simulink model "sample_trajectory"  (R2014a)
settings: Solver=ode3  StartTime=0.0  StopTime=2*apex_time  FixedStep=0.001  MaxStep=1e-2  RelTol=1e-3  AbsTol=1e-4
undefined symbols (not defined in the file or in its folder): alpha_apex, apex_time, d_y_com, l0_virtual, max_leg_length, min_leg_length
libraries: simulink x10
settings Model: Creator=wmartin  LastModifiedBy=wmartin

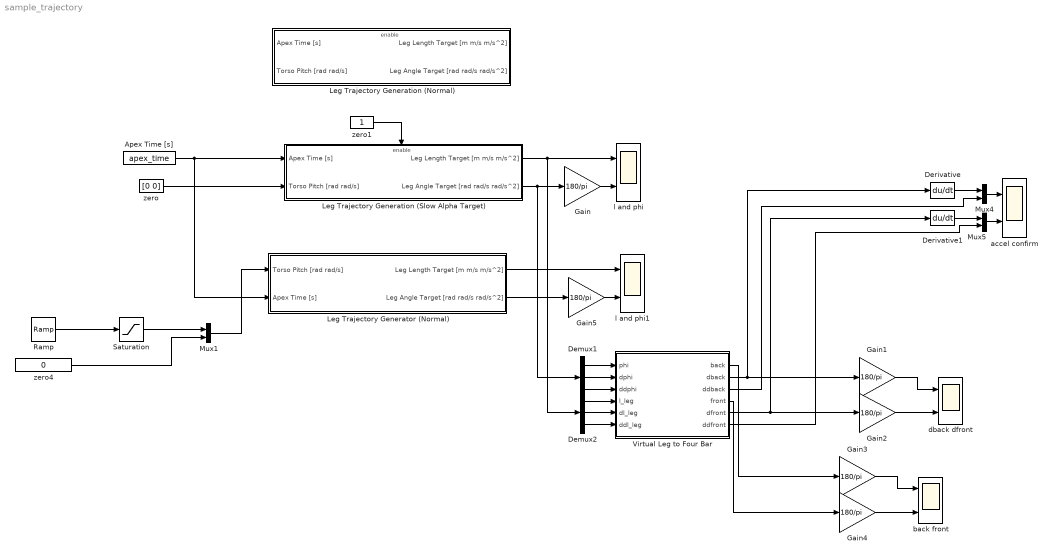
== system sample_trajectory ==
  Apex Time [s] : Constant  Value=apex_time
  Demux1 : Demux  Outputs=3
  Demux2 : Demux  Outputs=3
  Derivative : Derivative
  Derivative1 : Derivative
  Gain{,1..5} (6 alike) : Gain  Gain=180/pi
  Leg Trajectory Generation (Normal) : Subsystem
  Leg Trajectory Generation (Slow Alpha Target) : Subsystem
  Leg Trajectory Generator (Normal) : Subsystem
  Mux1 : Mux  Inputs=2
  Mux4 : Mux  Inputs=2
  Mux5 : Mux  Inputs=2
  Ramp : simulink/Sources/Ramp  slope=-20*pi/180 / apex_time  start=0  X0=0
  Saturation : Saturate  UpperLimit=20*pi/180  LowerLimit=-20*pi/180
  Virtual Leg to Four Bar : MATLAB Function  TreatAsAtomicUnit=on
  accel confirm : Scope  NumInputPorts=2
      settings: YMin=-5~-5  YMax=5~5  SaveName=ScopeData3
  back front : Scope  NumInputPorts=2
      settings: YMin=-5~-5  YMax=5~5  SaveName=ScopeData4
  dback dfront : Scope  NumInputPorts=2
      settings: YMin=-5~-5  YMax=5~5
  l and phi : Scope  NumInputPorts=2
      settings: YMin=-5~-5  YMax=5~5  SaveName=ScopeData2
  l and phi1 : Scope  NumInputPorts=2
      settings: YMin=-35~-3500  YMax=40~4000  SaveName=ScopeData5
  zero : Constant  Value=[0 0]
  zero1 : Constant
  zero4 : Constant  Value=0
  wires:
  Gain/1 -> l and phi/2
  Leg Trajectory Generation (Slow Alpha Target)/2(Leg Angle Target [rad rad/s rad/s^2]) -> Demux1/1, Gain/1
  Apex Time [s]/1 -> Leg Trajectory Generator (Normal)/2(Apex Time [s]), Leg Trajectory Generation (Slow Alpha Target)/1(Apex Time [s])
  Leg Trajectory Generation (Slow Alpha Target)/1(Leg Length Target [m m/s m/s^2]) -> Demux2/1, l and phi/1
  Demux1/1 -> Virtual Leg to Four Bar/1(phi)
  Demux1/2 -> Virtual Leg to Four Bar/2(dphi)
  Demux2/1 -> Virtual Leg to Four Bar/4(l_leg)
  Demux2/2 -> Virtual Leg to Four Bar/5(dl_leg)
  Gain1/1 -> dback dfront/1
  Gain2/1 -> dback dfront/2
  Virtual Leg to Four Bar/3(ddback) -> Mux4/2
  Virtual Leg to Four Bar/5(dfront) -> Derivative1/1, Gain2/1
  Virtual Leg to Four Bar/6(ddfront) -> Mux5/2
  Virtual Leg to Four Bar/2(dback) -> Derivative/1, Gain1/1
  Derivative/1 -> Mux4/1
  Mux4/1 -> accel confirm/1
  Derivative1/1 -> Mux5/1
  Mux5/1 -> accel confirm/2
  Demux1/3 -> Virtual Leg to Four Bar/3(ddphi)
  Demux2/3 -> Virtual Leg to Four Bar/6(ddl_leg)
  Gain3/1 -> back front/1
  Gain4/1 -> back front/2
  Virtual Leg to Four Bar/1(back) -> Gain3/1
  Virtual Leg to Four Bar/4(front) -> Gain4/1
  zero1/1 -> Leg Trajectory Generation (Slow Alpha Target)/Enable
  Gain5/1 -> l and phi1/2
  Leg Trajectory Generator (Normal)/1(Leg Length Target [m m/s m/s^2]) -> l and phi1/1
  Leg Trajectory Generator (Normal)/2(Leg Angle Target [rad rad/s rad/s^2]) -> Gain5/1
  zero/1 -> Leg Trajectory Generation (Slow Alpha Target)/2(Torso Pitch [rad rad/s])
  zero4/1 -> Mux1/2
  Mux1/1 -> Leg Trajectory Generator (Normal)/1(Torso Pitch [rad rad/s])
  Ramp/1 -> Saturation/1
  Saturation/1 -> Mux1/1

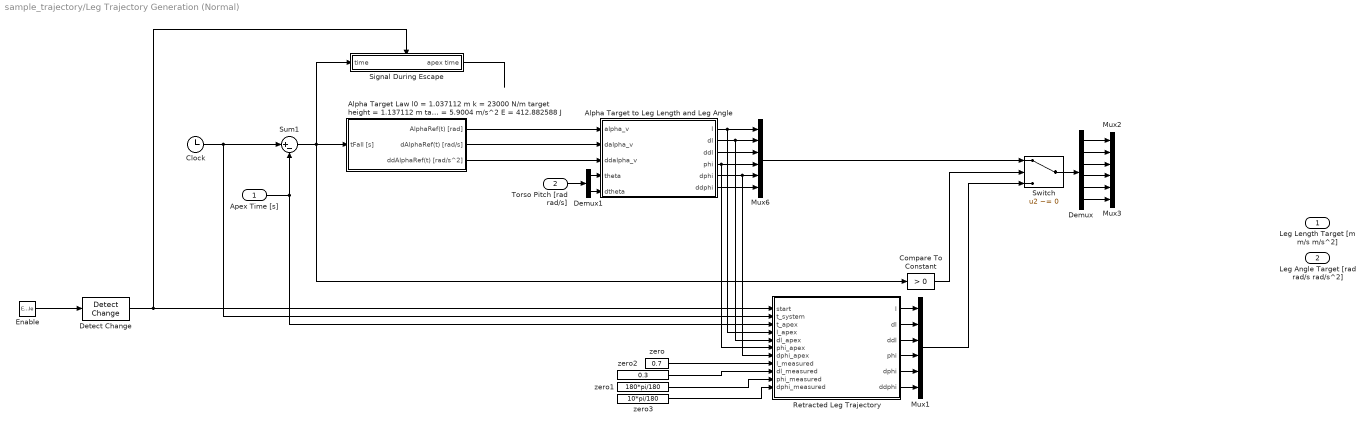
== system sample_trajectory/Leg Trajectory Generation (Normal) ==
  Apex Time [s] : Inport
  Torso Pitch [rad rad/s] : Inport  Port=2
  Enable : EnablePort  StatesWhenEnabling=reset  ShowOutputPort=on  ZeroCross=off
      settings: AttributesFormatString=When enabled: %<StatesWhenEnabling>
  Alpha Target Law l0 = 1.037112 m k = 23000 N/m target height = 1.137112 m target speed = 0.5 m/s m = 60.4120 kg g = 5.9004 m/s^2 E = 412.882588 J : Subsystem
  Alpha Target to Leg Length and Leg Angle : MATLAB Function  TreatAsAtomicUnit=on
  Clock : Clock
  Compare To Constant : simulink/Logic and Bit Operations/Compare To Constant  relop=>  const=0  OutDataTypeStr=boolean  ZeroCross=off
  Demux : Demux  Outputs=6
  Demux1 : Demux  Outputs=2
  Detect Change : simulink/Logic and Bit Operations/Detect Change  vinit=0  InputProcessing=Inherited  OutDataTypeStr=boolean
  Mux1 : Mux  Inputs=6
  Mux2 : Mux  Inputs=3
  Mux3 : Mux  Inputs=3
  Mux6 : Mux  Inputs=6
  Retracted Leg Trajectory : MATLAB Function  TreatAsAtomicUnit=on
  Signal During Escape : Subsystem
  Sum1 : Sum  Inputs=|+-
  Switch : Switch  Criteria=u2 ~= 0
  zero : Constant  Value=0.7
  zero1 : Constant  Value=180*pi/180
  zero2 : Constant  Value=0.3
  zero3 : Constant  Value=10*pi/180
  Leg Length Target [m m/s m/s^2] : Outport
  Leg Angle Target [rad rad/s rad/s^2] : Outport  Port=2
  wires:
  Signal During Escape/1(apex time) -> ?
  Clock/1 -> Sum1/1, Retracted Leg Trajectory/2(t_system)
  zero3/1 -> Retracted Leg Trajectory/11(dphi_measured)
  zero1/1 -> Retracted Leg Trajectory/10(phi_measured)
  zero2/1 -> Retracted Leg Trajectory/9(dl_measured)
  zero/1 -> Retracted Leg Trajectory/8(l_measured)
  Torso Pitch [rad rad/s]/1 -> Demux1/1
  Mux1/1 -> Switch/3
  Compare To Constant/1 -> Switch/2
  Apex Time [s]/1 -> Sum1/2, Retracted Leg Trajectory/3(t_apex)
  Alpha Target Law l0 = 1.037112 m k = 23000 N/m target height = 1.137112 m target speed = 0.5 m/s m = 60.4120 kg g = 5.9004 m/s^2 E = 412.882588 J/1(AlphaRef(t) [rad]) -> Alpha Target to Leg Length and Leg Angle/1(alpha_v)
  Sum1/1 -> Compare To Constant/1, Alpha Target Law l0 = 1.037112 m k = 23000 N/m target height = 1.137112 m target speed = 0.5 m/s m = 60.4120 kg g = 5.9004 m/s^2 E = 412.882588 J/1(tFall [s]), Signal During Escape/1(time)
  Retracted Leg Trajectory/1(l) -> Mux1/1
  Retracted Leg Trajectory/4(phi) -> Mux1/4
  Retracted Leg Trajectory/2(dl) -> Mux1/2
  Retracted Leg Trajectory/5(dphi) -> Mux1/5
  Enable/1 -> Detect Change/1
  Detect Change/1 -> Retracted Leg Trajectory/1(start), Signal During Escape/Enable
  Alpha Target to Leg Length and Leg Angle/4(phi) -> Mux6/4, Retracted Leg Trajectory/6(phi_apex)
  Alpha Target to Leg Length and Leg Angle/3(ddl) -> Mux6/3
  Alpha Target to Leg Length and Leg Angle/5(dphi) -> Mux6/5, Retracted Leg Trajectory/7(dphi_apex)
  Alpha Target to Leg Length and Leg Angle/6(ddphi) -> Mux6/6
  Alpha Target to Leg Length and Leg Angle/2(dl) -> Mux6/2, Retracted Leg Trajectory/5(dl_apex)
  Alpha Target to Leg Length and Leg Angle/1(l) -> Mux6/1, Retracted Leg Trajectory/4(l_apex)
  Switch/1 -> Demux/1
  Demux/6 -> Mux3/3
  Demux/5 -> Mux3/2
  Demux/4 -> Mux3/1
  Demux/3 -> Mux2/3
  Demux/2 -> Mux2/2
  Demux/1 -> Mux2/1
  Demux1/1 -> Alpha Target to Leg Length and Leg Angle/4(theta)
  Demux1/2 -> Alpha Target to Leg Length and Leg Angle/5(dtheta)
  Mux6/1 -> Switch/1
  Alpha Target Law l0 = 1.037112 m k = 23000 N/m target height = 1.137112 m target speed = 0.5 m/s m = 60.4120 kg g = 5.9004 m/s^2 E = 412.882588 J/3(ddAlphaRef(t) [rad/s^2]) -> Alpha Target to Leg Length and Leg Angle/3(ddalpha_v)
  Alpha Target Law l0 = 1.037112 m k = 23000 N/m target height = 1.137112 m target speed = 0.5 m/s m = 60.4120 kg g = 5.9004 m/s^2 E = 412.882588 J/2(dAlphaRef(t) [rad/s]) -> Alpha Target to Leg Length and Leg Angle/2(dalpha_v)
  Retracted Leg Trajectory/3(ddl) -> Mux1/3
  Retracted Leg Trajectory/6(ddphi) -> Mux1/6

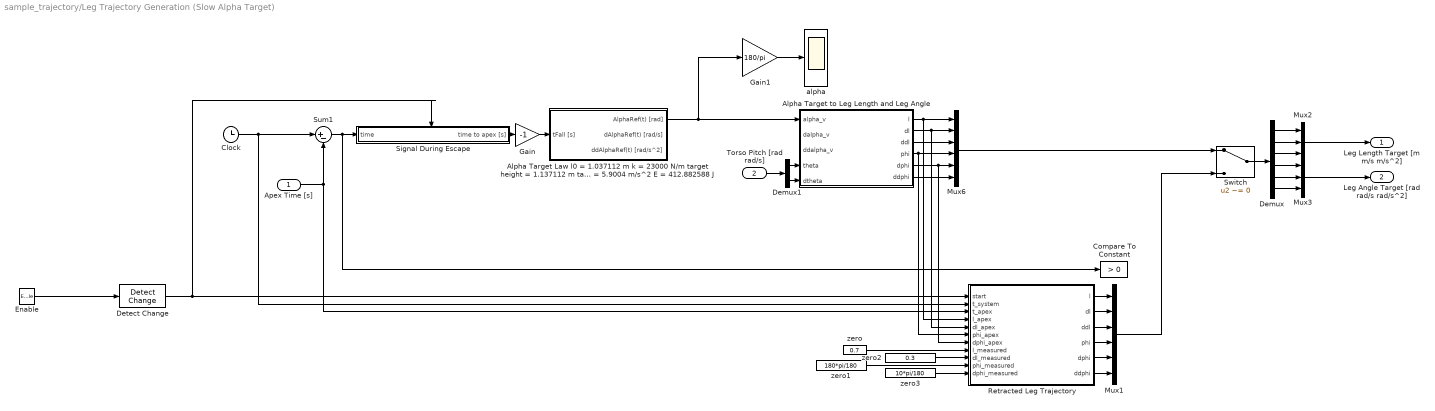
== system sample_trajectory/Leg Trajectory Generation (Slow Alpha Target) ==
  Apex Time [s] : Inport
  Torso Pitch [rad rad/s] : Inport  Port=2
  Enable : EnablePort  StatesWhenEnabling=reset  ShowOutputPort=on  ZeroCross=off
      settings: AttributesFormatString=When enabled: %<StatesWhenEnabling>
  Alpha Target Law l0 = 1.037112 m k = 23000 N/m target height = 1.137112 m target speed = 0.5 m/s m = 60.4120 kg g = 5.9004 m/s^2 E = 412.882588 J : Subsystem
  Alpha Target to Leg Length and Leg Angle : MATLAB Function  TreatAsAtomicUnit=on
  Clock : Clock
  Compare To Constant : simulink/Logic and Bit Operations/Compare To Constant  relop=>  const=0  OutDataTypeStr=boolean  ZeroCross=off
  Demux : Demux  Outputs=6
  Demux1 : Demux  Outputs=2
  Detect Change : simulink/Logic and Bit Operations/Detect Change  vinit=0  InputProcessing=Inherited  OutDataTypeStr=boolean
  Gain : Gain  Gain=-1
  Gain1 : Gain  Gain=180/pi
  Mux1 : Mux  Inputs=6
  Mux2 : Mux  Inputs=3
  Mux3 : Mux  Inputs=3
  Mux6 : Mux  Inputs=6
  Retracted Leg Trajectory : MATLAB Function  TreatAsAtomicUnit=on
  Signal During Escape : Subsystem
  Sum1 : Sum  Inputs=|+-
  Switch : Switch  Criteria=u2 ~= 0
  alpha : Scope
  zero : Constant  Value=0.7
  zero1 : Constant  Value=180*pi/180
  zero2 : Constant  Value=0.3
  zero3 : Constant  Value=10*pi/180
  Leg Length Target [m m/s m/s^2] : Outport
  Leg Angle Target [rad rad/s rad/s^2] : Outport  Port=2
  wires:
  Retracted Leg Trajectory/6(ddphi) -> Mux1/6
  Retracted Leg Trajectory/3(ddl) -> Mux1/3
  Mux6/1 -> Switch/1
  Demux1/2 -> Alpha Target to Leg Length and Leg Angle/5(dtheta)
  Demux1/1 -> Alpha Target to Leg Length and Leg Angle/4(theta)
  Demux/1 -> Mux2/1
  Demux/2 -> Mux2/2
  Demux/3 -> Mux2/3
  Demux/4 -> Mux3/1
  Demux/5 -> Mux3/2
  Demux/6 -> Mux3/3
  Switch/1 -> Demux/1
  Alpha Target to Leg Length and Leg Angle/1(l) -> Retracted Leg Trajectory/4(l_apex), Mux6/1
  Alpha Target to Leg Length and Leg Angle/2(dl) -> Retracted Leg Trajectory/5(dl_apex), Mux6/2
  Alpha Target to Leg Length and Leg Angle/6(ddphi) -> Mux6/6
  Alpha Target to Leg Length and Leg Angle/5(dphi) -> Retracted Leg Trajectory/7(dphi_apex), Mux6/5
  Alpha Target to Leg Length and Leg Angle/3(ddl) -> Mux6/3
  Alpha Target to Leg Length and Leg Angle/4(phi) -> Retracted Leg Trajectory/6(phi_apex), Mux6/4
  Detect Change/1 -> Retracted Leg Trajectory/1(start), Signal During Escape/Enable
  Apex Time [s]/1 -> Retracted Leg Trajectory/3(t_apex), Sum1/2
  Retracted Leg Trajectory/5(dphi) -> Mux1/5
  Retracted Leg Trajectory/2(dl) -> Mux1/2
  Retracted Leg Trajectory/4(phi) -> Mux1/4
  Retracted Leg Trajectory/1(l) -> Mux1/1
  Sum1/1 -> Signal During Escape/1(time), Compare To Constant/1
  Alpha Target Law l0 = 1.037112 m k = 23000 N/m target height = 1.137112 m target speed = 0.5 m/s m = 60.4120 kg g = 5.9004 m/s^2 E = 412.882588 J/1(AlphaRef(t) [rad]) -> Gain1/1, Alpha Target to Leg Length and Leg Angle/1(alpha_v)
  Mux1/1 -> Switch/3
  Torso Pitch [rad rad/s]/1 -> Demux1/1
  zero/1 -> Retracted Leg Trajectory/8(l_measured)
  zero2/1 -> Retracted Leg Trajectory/9(dl_measured)
  zero1/1 -> Retracted Leg Trajectory/10(phi_measured)
  zero3/1 -> Retracted Leg Trajectory/11(dphi_measured)
  Clock/1 -> Retracted Leg Trajectory/2(t_system), Sum1/1
  Signal During Escape/1(time to apex [s]) -> Gain/1
  Gain/1 -> Alpha Target Law l0 = 1.037112 m k = 23000 N/m target height = 1.137112 m target speed = 0.5 m/s m = 60.4120 kg g = 5.9004 m/s^2 E = 412.882588 J/1(tFall [s])
  Mux2/1 -> Leg Length Target [m m/s m/s^2]/1
  Mux3/1 -> Leg Angle Target [rad rad/s rad/s^2]/1
  Enable/1 -> Detect Change/1
  Gain1/1 -> alpha/1

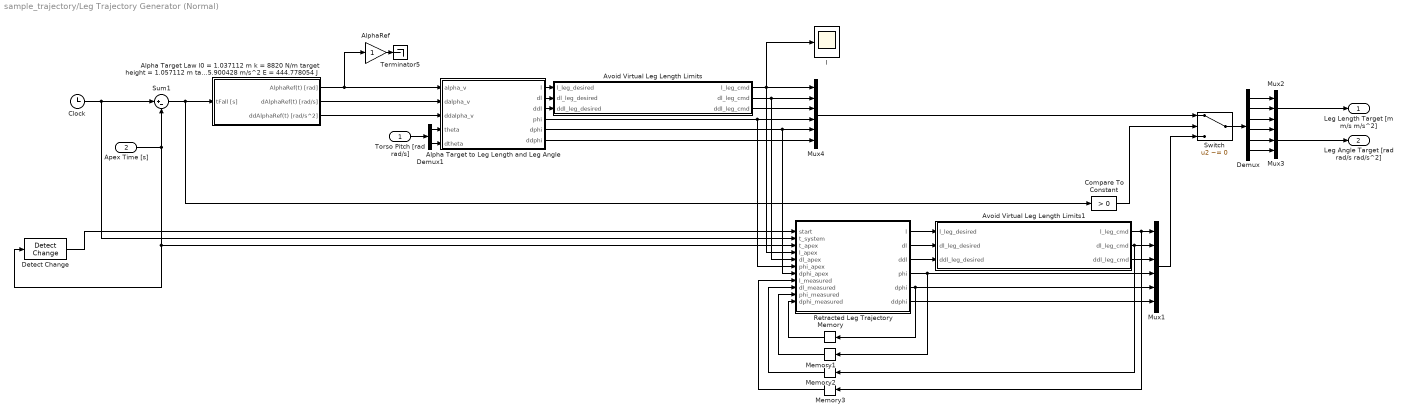
== system sample_trajectory/Leg Trajectory Generator (Normal) ==
  Torso Pitch [rad rad/s] : Inport
  Apex Time [s] : Inport  Port=2
  Alpha Target Law l0 = 1.037112 m k = 8820 N/m target height = 1.057112 m target speed = 1.0 m/s m = 60.4120 kg g = 5.900428 m/s^2 E = 444.778054 J : Subsystem
  Alpha Target to Leg Length and Leg Angle : MATLAB Function  TreatAsAtomicUnit=on
  AlphaRef : Gain
  Avoid Virtual Leg Length Limits : MATLAB Function  TreatAsAtomicUnit=on
  Avoid Virtual Leg Length Limits1 : MATLAB Function  TreatAsAtomicUnit=on
  Clock : Clock
  Compare To Constant : simulink/Logic and Bit Operations/Compare To Constant  relop=>  const=0  OutDataTypeStr=boolean  ZeroCross=off
  Demux : Demux  Outputs=6
  Demux1 : Demux  Outputs=2
  Detect Change : simulink/Logic and Bit Operations/Detect Change  vinit=0  InputProcessing=Inherited  OutDataTypeStr=boolean
  Memory : Memory  X0=-10*pi/180
  Memory1 : Memory  X0=159.2*pi/180
  Memory2 : Memory  X0=0.3
  Memory3 : Memory  X0=0.7738
  Mux1 : Mux  Inputs=6
  Mux2 : Mux  Inputs=3
  Mux3 : Mux  Inputs=3
  Mux4 : Mux  Inputs=6
  Retracted Leg Trajectory : MATLAB Function  TreatAsAtomicUnit=on
  Sum1 : Sum  Inputs=|+-
  Switch : Switch  Criteria=u2 ~= 0
  Terminator5 : Terminator
  l : Scope
      settings: SaveName=ScopeData6
  Leg Length Target [m m/s m/s^2] : Outport
  Leg Angle Target [rad rad/s rad/s^2] : Outport  Port=2
  wires:
  Torso Pitch [rad rad/s]/1 -> Demux1/1
  Mux1/1 -> Switch/3
  Compare To Constant/1 -> Switch/2
  Apex Time [s]/1 -> Detect Change/1, Retracted Leg Trajectory/3(t_apex), Sum1/2
  Clock/1 -> Retracted Leg Trajectory/2(t_system), Sum1/1
  Alpha Target Law l0 = 1.037112 m k = 8820 N/m target height = 1.057112 m target speed = 1.0 m/s m = 60.4120 kg g = 5.900428 m/s^2 E = 444.778054 J/1(AlphaRef(t) [rad]) -> AlphaRef/1, Alpha Target to Leg Length and Leg Angle/1(alpha_v)
  Sum1/1 -> Alpha Target Law l0 = 1.037112 m k = 8820 N/m target height = 1.057112 m target speed = 1.0 m/s m = 60.4120 kg g = 5.900428 m/s^2 E = 444.778054 J/1(tFall [s]), Compare To Constant/1
  AlphaRef/1 -> Terminator5/1
  Retracted Leg Trajectory/4(phi) -> Memory1/1, Mux1/4
  Retracted Leg Trajectory/5(dphi) -> Memory/1, Mux1/5
  Detect Change/1 -> Retracted Leg Trajectory/1(start)
  Alpha Target to Leg Length and Leg Angle/4(phi) -> Retracted Leg Trajectory/6(phi_apex), Mux4/4
  Avoid Virtual Leg Length Limits/2(dl_leg_cmd) -> Mux4/2, Retracted Leg Trajectory/5(dl_apex)
  Alpha Target to Leg Length and Leg Angle/5(dphi) -> Retracted Leg Trajectory/7(dphi_apex), Mux4/5
  Alpha Target to Leg Length and Leg Angle/6(ddphi) -> Mux4/6
  Avoid Virtual Leg Length Limits/1(l_leg_cmd) -> l/1, Mux4/1, Retracted Leg Trajectory/4(l_apex)
  Switch/1 -> Demux/1
  Mux2/1 -> Leg Length Target [m m/s m/s^2]/1
  Mux3/1 -> Leg Angle Target [rad rad/s rad/s^2]/1
  Demux/6 -> Mux3/3
  Demux/5 -> Mux3/2
  Demux/4 -> Mux3/1
  Demux/3 -> Mux2/3
  Demux/2 -> Mux2/2
  Demux/1 -> Mux2/1
  Demux1/1 -> Alpha Target to Leg Length and Leg Angle/4(theta)
  Demux1/2 -> Alpha Target to Leg Length and Leg Angle/5(dtheta)
  Mux4/1 -> Switch/1
  Alpha Target Law l0 = 1.037112 m k = 8820 N/m target height = 1.057112 m target speed = 1.0 m/s m = 60.4120 kg g = 5.900428 m/s^2 E = 444.778054 J/3(ddAlphaRef(t) [rad/s^2]) -> Alpha Target to Leg Length and Leg Angle/3(ddalpha_v)
  Alpha Target Law l0 = 1.037112 m k = 8820 N/m target height = 1.057112 m target speed = 1.0 m/s m = 60.4120 kg g = 5.900428 m/s^2 E = 444.778054 J/2(dAlphaRef(t) [rad/s]) -> Alpha Target to Leg Length and Leg Angle/2(dalpha_v)
  Retracted Leg Trajectory/6(ddphi) -> Mux1/6
  Avoid Virtual Leg Length Limits/3(ddl_leg_cmd) -> Mux4/3
  Alpha Target to Leg Length and Leg Angle/1(l) -> Avoid Virtual Leg Length Limits/1(l_leg_desired)
  Alpha Target to Leg Length and Leg Angle/2(dl) -> Avoid Virtual Leg Length Limits/2(dl_leg_desired)
  Alpha Target to Leg Length and Leg Angle/3(ddl) -> Avoid Virtual Leg Length Limits/3(ddl_leg_desired)
  Retracted Leg Trajectory/1(l) -> Avoid Virtual Leg Length Limits1/1(l_leg_desired)
  Retracted Leg Trajectory/2(dl) -> Avoid Virtual Leg Length Limits1/2(dl_leg_desired)
  Retracted Leg Trajectory/3(ddl) -> Avoid Virtual Leg Length Limits1/3(ddl_leg_desired)
  Avoid Virtual Leg Length Limits1/1(l_leg_cmd) -> Memory3/1, Mux1/1
  Avoid Virtual Leg Length Limits1/2(dl_leg_cmd) -> Memory2/1, Mux1/2
  Avoid Virtual Leg Length Limits1/3(ddl_leg_cmd) -> Mux1/3
  Memory/1 -> Retracted Leg Trajectory/11(dphi_measured)
  Memory1/1 -> Retracted Leg Trajectory/10(phi_measured)
  Memory2/1 -> Retracted Leg Trajectory/9(dl_measured)
  Memory3/1 -> Retracted Leg Trajectory/8(l_measured)

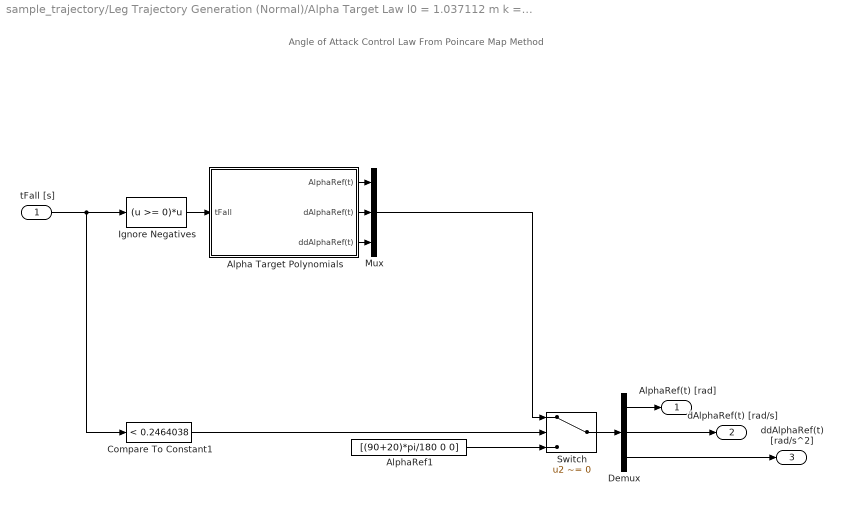
== system sample_trajectory/Leg Trajectory Generation (Normal)/Alpha Target Law l0 = 1.037112 m k = 23000 N//m target height = 1.137112 m target speed = 0.5 m//s m = 60.4120 kg g = 5.9004 m//s^2 E = 412.882588 J ==
  note: Angle of Attack Control Law From Poincare Map Method
  tFall [s] : Inport
  Alpha Target Polynomials : Subsystem
  AlphaRef1 : Constant  Value=[(90+20)*pi/180 0 0]
  Compare To Constant1 : simulink/Logic and Bit Operations/Compare To Constant  relop=<  const=0.2464038  OutDataTypeStr=boolean  ZeroCross=off
  Demux : Demux  Outputs=3
  Ignore Negatives : Fcn  Expr=(u >= 0)*u
  Mux : Mux  Inputs=3
  Switch : Switch  Criteria=u2 ~= 0
  AlphaRef(t) [rad] : Outport
  dAlphaRef(t) [rad/s] : Outport  Port=2
  ddAlphaRef(t) [rad/s^2] : Outport  Port=3
  wires:
  Ignore Negatives/1 -> Alpha Target Polynomials/1(tFall)
  Mux/1 -> Switch/1
  Alpha Target Polynomials/1(AlphaRef(t)) -> Mux/1
  Alpha Target Polynomials/3(ddAlphaRef(t)) -> Mux/3
  Alpha Target Polynomials/2(dAlphaRef(t)) -> Mux/2
  Compare To Constant1/1 -> Switch/2
  tFall [s]/1 -> Compare To Constant1/1, Ignore Negatives/1
  Switch/1 -> Demux/1
  Demux/1 -> AlphaRef(t) [rad]/1
  Demux/2 -> dAlphaRef(t) [rad/s]/1
  Demux/3 -> ddAlphaRef(t) [rad/s^2]/1
  AlphaRef1/1 -> Switch/3

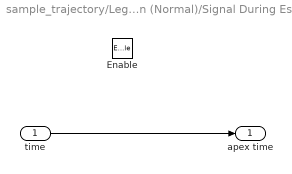
== system sample_trajectory/Leg Trajectory Generation (Normal)/Signal During Escape ==
  time : Inport
  Enable : EnablePort
  apex time : Outport
  wires:
  time/1 -> apex time/1

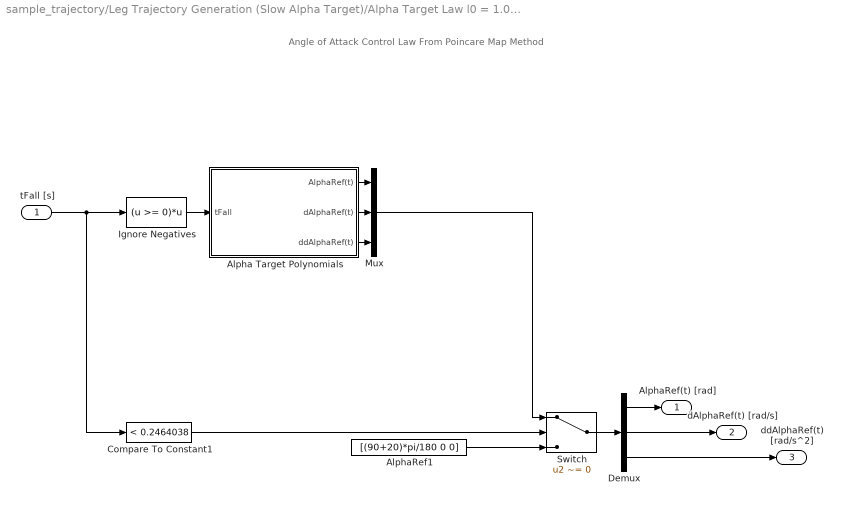
== system sample_trajectory/Leg Trajectory Generation (Slow Alpha Target)/Alpha Target Law l0 = 1.037112 m k = 23000 N//m target height = 1.137112 m target speed = 0.5 m//s m = 60.4120 kg g = 5.9004 m//s^2 E = 412.882588 J ==
  note: Angle of Attack Control Law From Poincare Map Method
  tFall [s] : Inport
  Alpha Target Polynomials : Subsystem
  AlphaRef1 : Constant  Value=[(90+20)*pi/180 0 0]
  Compare To Constant1 : simulink/Logic and Bit Operations/Compare To Constant  relop=<  const=0.2464038  OutDataTypeStr=boolean  ZeroCross=off
  Demux : Demux  Outputs=3
  Ignore Negatives : Fcn  Expr=(u >= 0)*u
  Mux : Mux  Inputs=3
  Switch : Switch  Criteria=u2 ~= 0
  AlphaRef(t) [rad] : Outport
  dAlphaRef(t) [rad/s] : Outport  Port=2
  ddAlphaRef(t) [rad/s^2] : Outport  Port=3
  wires:
  AlphaRef1/1 -> Switch/3
  Demux/3 -> ddAlphaRef(t) [rad/s^2]/1
  Demux/2 -> dAlphaRef(t) [rad/s]/1
  Demux/1 -> AlphaRef(t) [rad]/1
  Switch/1 -> Demux/1
  tFall [s]/1 -> Ignore Negatives/1, Compare To Constant1/1
  Compare To Constant1/1 -> Switch/2
  Alpha Target Polynomials/2(dAlphaRef(t)) -> Mux/2
  Alpha Target Polynomials/3(ddAlphaRef(t)) -> Mux/3
  Alpha Target Polynomials/1(AlphaRef(t)) -> Mux/1
  Mux/1 -> Switch/1
  Ignore Negatives/1 -> Alpha Target Polynomials/1(tFall)

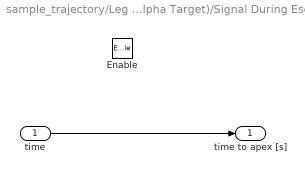
== system sample_trajectory/Leg Trajectory Generation (Slow Alpha Target)/Signal During Escape ==
  time : Inport
  Enable : EnablePort
  time to apex [s] : Outport
  wires:
  time/1 -> time to apex [s]/1

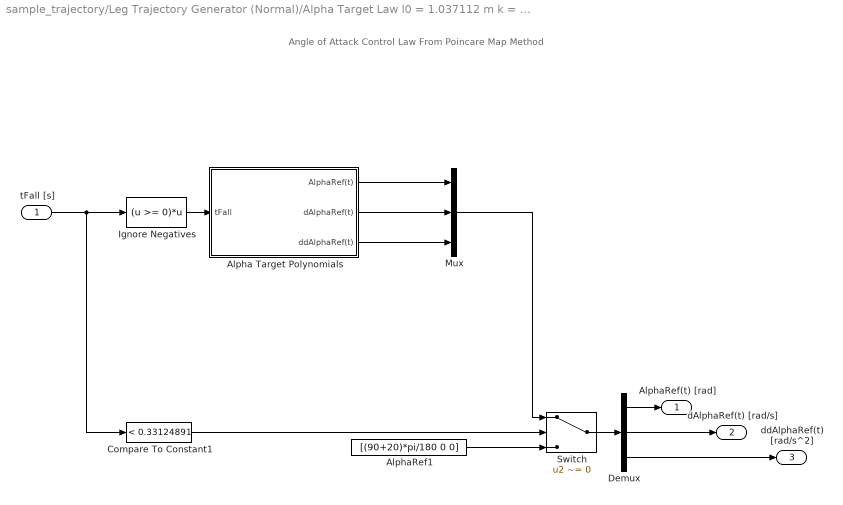
== system sample_trajectory/Leg Trajectory Generator (Normal)/Alpha Target Law l0 = 1.037112 m k = 8820 N//m target height = 1.057112 m target speed = 1.0 m//s m = 60.4120 kg g = 5.900428 m//s^2 E = 444.778054 J ==
  note: Angle of Attack Control Law From Poincare Map Method
  tFall [s] : Inport
  Alpha Target Polynomials : Subsystem
  AlphaRef1 : Constant  Value=[(90+20)*pi/180 0 0]
  Compare To Constant1 : simulink/Logic and Bit Operations/Compare To Constant  relop=<  const=0.33124891  OutDataTypeStr=boolean  ZeroCross=off
  Demux : Demux  Outputs=3
  Ignore Negatives : Fcn  Expr=(u >= 0)*u
  Mux : Mux  Inputs=3
  Switch : Switch  Criteria=u2 ~= 0
  AlphaRef(t) [rad] : Outport
  dAlphaRef(t) [rad/s] : Outport  Port=2
  ddAlphaRef(t) [rad/s^2] : Outport  Port=3
  wires:
  Alpha Target Polynomials/1(AlphaRef(t)) -> Mux/1
  AlphaRef1/1 -> Switch/3
  Demux/3 -> ddAlphaRef(t) [rad/s^2]/1
  Demux/2 -> dAlphaRef(t) [rad/s]/1
  Demux/1 -> AlphaRef(t) [rad]/1
  Switch/1 -> Demux/1
  tFall [s]/1 -> Ignore Negatives/1, Compare To Constant1/1
  Compare To Constant1/1 -> Switch/2
  Alpha Target Polynomials/2(dAlphaRef(t)) -> Mux/2
  Alpha Target Polynomials/3(ddAlphaRef(t)) -> Mux/3
  Mux/1 -> Switch/1
  Ignore Negatives/1 -> Alpha Target Polynomials/1(tFall)

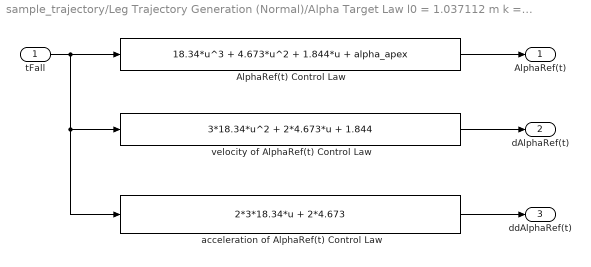
== system sample_trajectory/Leg Trajectory Generation (Normal)/Alpha Target Law l0 = 1.037112 m k = 23000 N//m target height = 1.137112 m target speed = 0.5 m//s m = 60.4120 kg g = 5.9004 m//s^2 E = 412.882588 J/Alpha Target Polynomials ==
  tFall : Inport
  AlphaRef(t) Control Law : Fcn  Expr=18.34*u^3 + 4.673*u^2 + 1.844*u + alpha_apex
  acceleration of AlphaRef(t) Control Law : Fcn  Expr=2*3*18.34*u + 2*4.673
  velocity of AlphaRef(t) Control Law : Fcn  Expr=3*18.34*u^2 + 2*4.673*u + 1.844
  AlphaRef(t) : Outport  OutputWhenDisabled=reset  InitialOutput=0
      settings: AttributesFormatString=When disabled: %<OutputWhenDisabled>\nDisabled Output: %<InitialOutput>
  dAlphaRef(t) : Outport  Port=2  OutputWhenDisabled=reset  InitialOutput=0
      settings: AttributesFormatString=When disbaled: %<OutputWhenDisabled>\nDisabled output: %<InitialOutput>
  ddAlphaRef(t) : Outport  Port=3  OutputWhenDisabled=reset  InitialOutput=0
      settings: AttributesFormatString=When disabled: %<OutputWhenDisabled>\nDisabled output: %<InitialOutput>
  wires:
  tFall/1 -> AlphaRef(t) Control Law/1, velocity of AlphaRef(t) Control Law/1, acceleration of AlphaRef(t) Control Law/1
  AlphaRef(t) Control Law/1 -> AlphaRef(t)/1
  velocity of AlphaRef(t) Control Law/1 -> dAlphaRef(t)/1
  acceleration of AlphaRef(t) Control Law/1 -> ddAlphaRef(t)/1

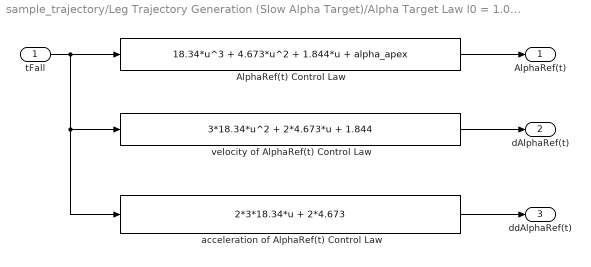
== system sample_trajectory/Leg Trajectory Generation (Slow Alpha Target)/Alpha Target Law l0 = 1.037112 m k = 23000 N//m target height = 1.137112 m target speed = 0.5 m//s m = 60.4120 kg g = 5.9004 m//s^2 E = 412.882588 J/Alpha Target Polynomials ==
  tFall : Inport
  AlphaRef(t) Control Law : Fcn  Expr=18.34*u^3 + 4.673*u^2 + 1.844*u + alpha_apex
  acceleration of AlphaRef(t) Control Law : Fcn  Expr=2*3*18.34*u + 2*4.673
  velocity of AlphaRef(t) Control Law : Fcn  Expr=3*18.34*u^2 + 2*4.673*u + 1.844
  AlphaRef(t) : Outport  OutputWhenDisabled=reset  InitialOutput=0
      settings: AttributesFormatString=When disabled: %<OutputWhenDisabled>\nDisabled Output: %<InitialOutput>
  dAlphaRef(t) : Outport  Port=2  OutputWhenDisabled=reset  InitialOutput=0
      settings: AttributesFormatString=When disbaled: %<OutputWhenDisabled>\nDisabled output: %<InitialOutput>
  ddAlphaRef(t) : Outport  Port=3  OutputWhenDisabled=reset  InitialOutput=0
      settings: AttributesFormatString=When disabled: %<OutputWhenDisabled>\nDisabled output: %<InitialOutput>
  wires:
  acceleration of AlphaRef(t) Control Law/1 -> ddAlphaRef(t)/1
  velocity of AlphaRef(t) Control Law/1 -> dAlphaRef(t)/1
  AlphaRef(t) Control Law/1 -> AlphaRef(t)/1
  tFall/1 -> acceleration of AlphaRef(t) Control Law/1, velocity of AlphaRef(t) Control Law/1, AlphaRef(t) Control Law/1

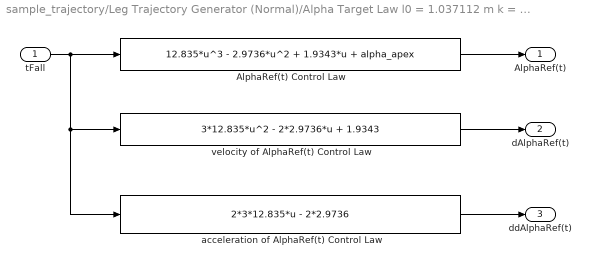
== system sample_trajectory/Leg Trajectory Generator (Normal)/Alpha Target Law l0 = 1.037112 m k = 8820 N//m target height = 1.057112 m target speed = 1.0 m//s m = 60.4120 kg g = 5.900428 m//s^2 E = 444.778054 J/Alpha Target Polynomials ==
  tFall : Inport
  AlphaRef(t) Control Law : Fcn  Expr=12.835*u^3 - 2.9736*u^2 + 1.9343*u + alpha_apex
  acceleration of AlphaRef(t) Control Law : Fcn  Expr=2*3*12.835*u - 2*2.9736
  velocity of AlphaRef(t) Control Law : Fcn  Expr=3*12.835*u^2 - 2*2.9736*u + 1.9343
  AlphaRef(t) : Outport  OutputWhenDisabled=reset  InitialOutput=0
      settings: AttributesFormatString=When disabled: %<OutputWhenDisabled>\nDisabled Output: %<InitialOutput>
  dAlphaRef(t) : Outport  Port=2  OutputWhenDisabled=reset  InitialOutput=0
      settings: AttributesFormatString=When disbaled: %<OutputWhenDisabled>\nDisabled output: %<InitialOutput>
  ddAlphaRef(t) : Outport  Port=3  OutputWhenDisabled=reset  InitialOutput=0
      settings: AttributesFormatString=When disabled: %<OutputWhenDisabled>\nDisabled output: %<InitialOutput>
  wires:
  acceleration of AlphaRef(t) Control Law/1 -> ddAlphaRef(t)/1
  velocity of AlphaRef(t) Control Law/1 -> dAlphaRef(t)/1
  AlphaRef(t) Control Law/1 -> AlphaRef(t)/1
  tFall/1 -> acceleration of AlphaRef(t) Control Law/1, velocity of AlphaRef(t) Control Law/1, AlphaRef(t) Control Law/1

== matlab function sample_trajectory/Leg Trajectory Generation (Normal)/Alpha Target to Leg Length and Leg Angle ==
  data: alpha_v input; dalpha_v input; ddalpha_v input; theta input; dtheta input; l output; dl output; ddl output; phi output; d_y_com parameter; l0_virtual parameter; dphi output; ddphi output
function [l, dl, ddl, phi, dphi, ddphi] = fcn(alpha_v, dalpha_v, ddalpha_v, theta, dtheta, d_y_com, l0_virtual)
    [l, dl, ddl, phi, dphi, ddphi] = AlphaTargetToVirtualLeg2D(alpha_v, dalpha_v, ddalpha_v, theta, dtheta, 0, d_y_com, l0_virtual);
end

== matlab function sample_trajectory/Virtual Leg to Four Bar ==
  data: phi input; dphi input; ddphi input; l_leg input; dl_leg input; back output; dback output; ddback output; front output; dfront output; ddl_leg input; ddfront output
function [back, dback, ddback, front, dfront, ddfront] = fcn(phi, dphi, ddphi, l_leg, dl_leg, ddl_leg)

    back  = phi + acos(l_leg);
    front = phi - acos(l_leg);
    
    dback  = dphi - dl_leg/sin((back-front)/2);
    dfront = dphi + dl_leg/sin((back-front)/2);
    
    ddback = ddphi - ddl_leg/(1 - l_leg^2)^(1/2) - (l_leg*dl_leg^2)/(1 - l_leg^2)^(3/2);
    ddfront = ddl_leg/(1 - l_leg^2)^(1/2) + ddphi + (l_leg*dl_leg^2)/(1 - l_leg^2)^(3/2);
    
end

== matlab function sample_trajectory/Leg Trajectory Generation (Normal)/Retracted Leg Trajectory ==
  data: start input; t_system input; t_apex input; l_apex input; dl_apex input; phi_apex input; dphi_apex input; l_measured input; dl_measured input; phi_measured input; l output; dl output; ddl output; phi output; dphi output; ddphi output; dphi_measured input
%% Generates a dynamically feasible trajectory for swinging the virtual leg between two points.
% Constrains to starting/ending positions and velocities.
% Minimizes torque squared
% May want to generate the trajectory in fourbar coordinates instead.
function [l, dl, ddl, phi, dphi, ddphi] = fcn(start, t_system, t_apex, l_apex, dl_apex, phi_apex, dphi_apex, l_measured, dl_measured, phi_measured, dphi_measured)

    persistent t_start l_start phi_start dl_start dphi_start;
    if isempty(t_start) || start
        t_start = t_system;
        l_start = l_measured;
        dl_start = dl_measured;
        phi_start = phi_measured;
        dphi_start = dphi_measured;
    end
    
    t = t_system - t_start;
    time_to_apex = t_apex - t_start;
    t = min(time_to_apex, t);

    % Virtual Leg Length
    [a0, a1, a2, a3] = ThirdOrderTrajectory(l_start, dl_start, l_apex, dl_apex, time_to_apex);
    l = a3*t^3 + a2*t^2 + a1*t + a0;
    dl = 3*a3*t^2 + 2*a2*t + a1;
    ddl = 6*a3*t + 2*a2;
    
    % Virtual Leg Angle
    [a0, a1, a2, a3] = ThirdOrderTrajectory(phi_start, dphi_start, phi_apex, dphi_apex, time_to_apex);
    phi = a3*t^3 + a2*t^2 + a1*t + a0;
    dphi = 3*a3*t^2 + 2*a2*t + a1;
    ddphi = 6*a3*t + 2*a2;

end

== matlab function sample_trajectory/Leg Trajectory Generator (Normal)/Alpha Target to Leg Length and Leg Angle ==
  data: alpha_v input; dalpha_v input; ddalpha_v input; theta input; dtheta input; l output; dl output; ddl output; phi output; d_y_com parameter; l0_virtual parameter; dphi output; ddphi output
function [l, dl, ddl, phi, dphi, ddphi] = fcn(alpha_v, dalpha_v, ddalpha_v, theta, dtheta, d_y_com, l0_virtual)
    [l, dl, ddl, phi, dphi, ddphi] = AlphaTargetToVirtualLeg2D(alpha_v, dalpha_v, ddalpha_v, theta, dtheta, 0, d_y_com, l0_virtual);
end

== matlab function sample_trajectory/Leg Trajectory Generator (Normal)/Retracted Leg Trajectory ==
  data: start input boolean; t_system input double; t_apex input double; l_apex input double; dl_apex input double; phi_apex input double; dphi_apex input double; l_measured input double; dl_measured input double; phi_measured input double; l output double; dl output double; ddl output double; phi output double; dphi output double; ddphi output double; dphi_measured input double
%% Generates a dynamically feasible trajectory for swinging the virtual leg between two points.
% Constrains to starting/ending positions and velocities.
% Minimizes torque squared
% May want to generate the trajectory in fourbar coordinates instead.
function [l, dl, ddl, phi, dphi, ddphi] = fcn(start, t_system, t_apex, l_apex, dl_apex, phi_apex, dphi_apex, l_measured, dl_measured, phi_measured, dphi_measured)

    persistent t_start l_start phi_start dl_start dphi_start;
    if isempty(t_start)
        t_start = t_system;
        l_start = l_measured;
        dl_start = dl_measured;
        phi_start = phi_measured;
        dphi_start = dphi_measured;
    end
    if start || (t_system - t_start) > 0.030
        t_start = t_system;
        l_start = l_measured;
        dl_start = dl_measured;
        phi_start = phi_measured;
        dphi_start = dphi_measured;
    end
    
    t = t_system - t_start;
    time_to_apex = t_apex - t_start;
    t = min(time_to_apex, t);

    % Virtual Leg Length
    [a0, a1, a2, a3] = ThirdOrderTrajectory(l_start, dl_start, l_apex, dl_apex, time_to_apex);
    l = a3*t^3 + a2*t^2 + a1*t + a0;
    dl = 3*a3*t^2 + 2*a2*t + a1;
    ddl = 6*a3*t + 2*a2;
    
    % Virtual Leg Angle
    [a0, a1, a2, a3] = ThirdOrderTrajectory(phi_start, dphi_start, phi_apex, dphi_apex, time_to_apex);
    phi = a3*t^3 + a2*t^2 + a1*t + a0;
    dphi = 3*a3*t^2 + 2*a2*t + a1;
    ddphi = 6*a3*t + 2*a2;

end

== matlab function sample_trajectory/Leg Trajectory Generator (Normal)/Avoid Virtual Leg Length Limits ==
  data: l_leg_desired input; dl_leg_desired input; ddl_leg_desired input; l_leg_cmd output double; dl_leg_cmd output double; ddl_leg_cmd output double; min_leg_length parameter; max_leg_length parameter
%% Avoid virtual leg length limits by ensuring we don't command position/velocities/accelerations that would hit them.
function [l_leg_cmd, dl_leg_cmd, ddl_leg_cmd] = AvoidVirtualLengthLimits(l_leg_desired, dl_leg_desired, ddl_leg_desired, min_leg_length, max_leg_length)
    [l_leg_cmd, dl_leg_cmd, ddl_leg_cmd] = AvoidVirtualLengthLimits(l_leg_desired, dl_leg_desired, ddl_leg_desired, min_leg_length, max_leg_length);
end

== matlab function sample_trajectory/Leg Trajectory Generator (Normal)/Avoid Virtual Leg Length Limits1 ==
  data: l_leg_desired input; dl_leg_desired input; ddl_leg_desired input; l_leg_cmd output double; dl_leg_cmd output double; ddl_leg_cmd output double; min_leg_length parameter; max_leg_length parameter
%% Avoid virtual leg length limits by ensuring we don't command position/velocities/accelerations that would hit them.
function [l_leg_cmd, dl_leg_cmd, ddl_leg_cmd] = AvoidVirtualLengthLimits(l_leg_desired, dl_leg_desired, ddl_leg_desired, min_leg_length, max_leg_length)
    [l_leg_cmd, dl_leg_cmd, ddl_leg_cmd] = AvoidVirtualLengthLimits(l_leg_desired, dl_leg_desired, ddl_leg_desired, min_leg_length, max_leg_length);
end

== matlab function sample_trajectory/Leg Trajectory Generation (Slow Alpha Target)/Alpha Target to Leg Length and Leg Angle ==
  data: alpha_v input; dalpha_v input; ddalpha_v input; theta input; dtheta input; l output; dl output; ddl output; phi output; d_y_com parameter; l0_virtual parameter; dphi output; ddphi output
function [l, dl, ddl, phi, dphi, ddphi] = fcn(alpha_v, dalpha_v, ddalpha_v, theta, dtheta, d_y_com, l0_virtual)
    [l, dl, ddl, phi, dphi, ddphi] = AlphaTargetToVirtualLeg2D(alpha_v, dalpha_v, ddalpha_v, theta, dtheta, 0, d_y_com, l0_virtual);
end

== matlab function sample_trajectory/Leg Trajectory Generation (Slow Alpha Target)/Retracted Leg Trajectory ==
  data: start input; t_system input; t_apex input; l_apex input; dl_apex input; phi_apex input; dphi_apex input; l_measured input; dl_measured input; phi_measured input; l output; dl output; ddl output; phi output; dphi output; ddphi output; dphi_measured input
%% Generates a dynamically feasible trajectory for swinging the virtual leg between two points.
% Constrains to starting/ending positions and velocities.
% Minimizes torque squared
% May want to generate the trajectory in fourbar coordinates instead.
function [l, dl, ddl, phi, dphi, ddphi] = fcn(start, t_system, t_apex, l_apex, dl_apex, phi_apex, dphi_apex, l_measured, dl_measured, phi_measured, dphi_measured)

    persistent t_start l_start phi_start dl_start dphi_start;
    if isempty(t_start) || start
        t_start = t_system;
        l_start = l_measured;
        dl_start = dl_measured;
        phi_start = phi_measured;
        dphi_start = dphi_measured;
    end
    
    t = t_system - t_start;
    time_to_apex = 2*(t_apex - t_start);
    t = min(time_to_apex, t);

    % Virtual Leg Length
    [a0, a1, a2, a3] = ThirdOrderTrajectory(l_start, dl_start, l_apex, dl_apex, time_to_apex);
    l = a3*t^3 + a2*t^2 + a1*t + a0;
    dl = 3*a3*t^2 + 2*a2*t + a1;
    ddl = 6*a3*t + 2*a2;
    
    % Virtual Leg Angle
    [a0, a1, a2, a3] = ThirdOrderTrajectory(phi_start, dphi_start, phi_apex, dphi_apex, time_to_apex);
    phi = a3*t^3 + a2*t^2 + a1*t + a0;
    dphi = 3*a3*t^2 + 2*a2*t + a1;
    ddphi = 6*a3*t + 2*a2;

end
